simulink library "testbench_lib"  (Simulink 6.2)
libraries: xbsIndex_r3 x4, casper_library x2
settings Model: LastModifiedBy=Glenn

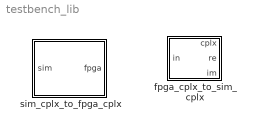
== system testbench_lib ==
  fpga_cplx_to_sim_cplx : Subsystem  mask{width=18}
      mask prompts: width "Data Width"
      mask help: Converts a Casper complex to a Simulink complex
      mask init:
      | set_param(gcb, 'AttributesFormatString', sprintf('%d_%d bit',width,width-1));
      settings: AttributesFormatString=18_17 bit
  sim_cplx_to_fpga_cplx : Subsystem  mask{width=18}
      mask prompts: width "Data Width"
      mask help:
      | Converts a Simulink complex to fixed point and concatenates it to a Casper complex.
      | Output is two Fix_width_(width-1) numbers concatenated.
      mask init:
      | set_param(gcb, 'AttributesFormatString', sprintf('%d_%d bit',width,width-1));
      settings: AttributesFormatString=18_17 bit

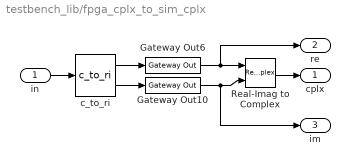
== system testbench_lib/fpga_cplx_to_sim_cplx ==
  in : Inport  Port=1  LatchInput=off
  Gateway Out10 : xbsIndex_r3/Gateway Out  output_type=Double  nbits=8  bin_pt=6  arith_type=Boolean  quantization=Truncate  overflow=Wrap  hdl_port=on  timing_constraint=None  locs_specified=off  LOCs={}  needs_fixed_name=off  show_param=off
      settings: xl_area=[0, 0, 0, 0, 0, 0, 0]
  Gateway Out6 : xbsIndex_r3/Gateway Out  output_type=Double  nbits=8  bin_pt=6  arith_type=Boolean  quantization=Truncate  overflow=Wrap  hdl_port=on  timing_constraint=None  locs_specified=off  LOCs={}  needs_fixed_name=off  show_param=off
      settings: xl_area=[0, 0, 0, 0, 0, 0, 0]
  Real-Imag to Complex : RealImagToComplex
  c_to_ri : casper_library/Misc/c_to_ri  n_bits=width  bin_pt=width-1
      settings: AttributesFormatString=49_56 r/i48_55 r/i
  cplx : Outport
  re : Outport  Port=2
  im : Outport  Port=3
  wires:
  in/1 -> c_to_ri/1
  Real-Imag to Complex/1 -> cplx/1
  Gateway Out10/1 -> im/1, Real-Imag to Complex/2
  Gateway Out6/1 -> re/1, Real-Imag to Complex/1
  c_to_ri/2 -> Gateway Out10/1
  c_to_ri/1 -> Gateway Out6/1

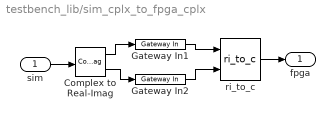
== system testbench_lib/sim_cplx_to_fpga_cplx ==
  sim : Inport  Port=1  LatchInput=off
  Complex to Real-Imag : ComplexToRealImag
  Gateway In1 : xbsIndex_r3/Gateway In  arith_type="Signed  (2's comp)"  n_bits=width  bin_pt=width-1  quantization=Truncate  overflow=Wrap  period=1  timing_constraint=None  locs_specified=off  LOCs={}  needs_fixed_name=off  dbl_ovrd=off  show_param=off
      settings: xl_area=[0, 0, 0, 0, 0, 0, 0]
  Gateway In2 : xbsIndex_r3/Gateway In  arith_type="Signed  (2's comp)"  n_bits=width  bin_pt=width-1  quantization=Truncate  overflow=Wrap  period=1  timing_constraint=None  locs_specified=off  LOCs={}  needs_fixed_name=off  dbl_ovrd=off  show_param=off
      settings: xl_area=[0, 0, 0, 0, 0, 0, 0]
  ri_to_c : casper_library/Misc/ri_to_c
  fpga : Outport
  wires:
  sim/1 -> Complex to Real-Imag/1
  ri_to_c/1 -> fpga/1
  Gateway In2/1 -> ri_to_c/2
  Gateway In1/1 -> ri_to_c/1
  Complex to Real-Imag/2 -> Gateway In2/1
  Complex to Real-Imag/1 -> Gateway In1/1
